simulink model "M"  (R2014a)
settings: Solver=ode45  StartTime=0.0  StopTime=1.0  RelTol=1e-3
undefined symbols (not defined in the file): DiscIntNeverNeededParam, find_system
libraries: powerlib x49, powerlib_extras x39, simulink_extras x4, simulink x2
(part 1 of 4)
settings Model: Creator=HP  LastModifiedBy=HP

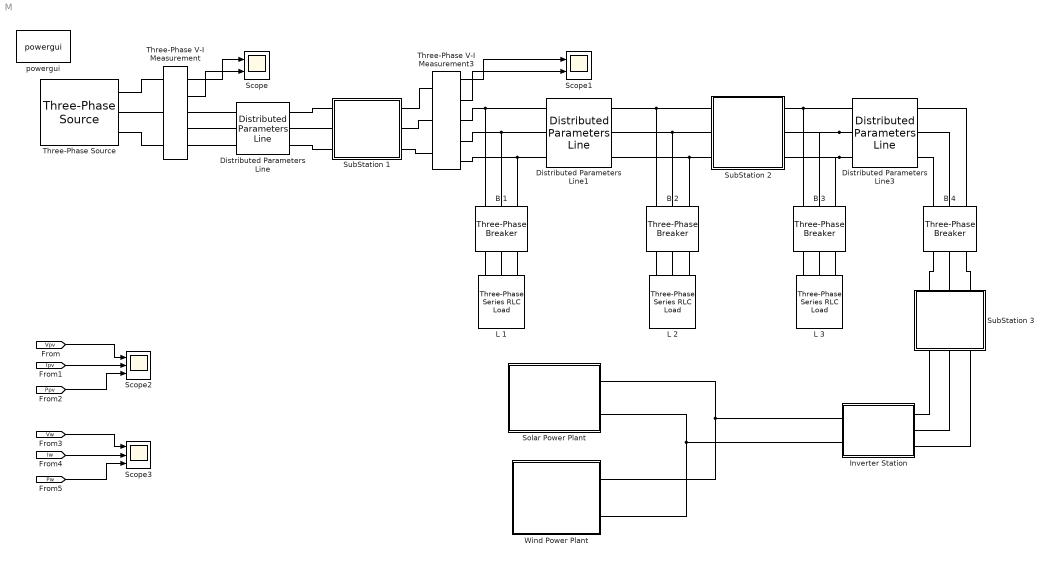
== system M ==
  B 1 : powerlib/Elements/Three-Phase Breaker  InitialState=closed  SwitchA=off  SwitchB=off  SwitchC=off  SwitchTimes="[0.02  0.4]"  External=off  BreakerResistance=0.001  SnubberResistance=1e6  SnubberCapacitance=inf  Measurements=None
  B 2 : powerlib/Elements/Three-Phase Breaker  InitialState=closed  SwitchA=off  SwitchB=off  SwitchC=off  SwitchTimes=[0.001 0.3]  External=off  BreakerResistance=0.001  SnubberResistance=1e6  SnubberCapacitance=inf  Measurements=None
  B 3 : powerlib/Elements/Three-Phase Breaker  InitialState=closed  SwitchA=off  SwitchB=off  SwitchC=off  SwitchTimes="[0.02  0.4]"  External=off  BreakerResistance=0.001  SnubberResistance=1e6  SnubberCapacitance=inf  Measurements=None
  B 4 : powerlib/Elements/Three-Phase Breaker  InitialState=closed  SwitchA=off  SwitchB=off  SwitchC=off  SwitchTimes="[0.001  0.3]"  External=off  BreakerResistance=0.001  SnubberResistance=1e6  SnubberCapacitance=inf  Measurements=None
  Distributed Parameters Line : powerlib/Elements/Distributed Parameters Line  Phases=3  Frequency=50  Resistance=[0.01273 0.3864]  Inductance="[0.9337e-3  4.1264e-3]"  Capacitance=[12.74e-9 7.751e-9]  Length=100  x1=[-0.0006 -7.49436978847816e-10 8343.24139426933 -24001.7141670507;-0.00055 -7.41002543974675e-10 8719.21464973306 -23867.7031951491;-0.0005 -7.32385277811667e-10 9093.03656945038 -23727.8032246242;-0.00045 -7.23587306540276e-10 9464.61491845621 -23582.0487737004;-0.0004 -7.14610800928265e-10 9833.85801535299 -23430.4758051074;-0.00035 -7.05457975794076e-10 10200.6747549317 -23273.1217172073;-0.0003 -6.96131089460354e-10 10564.9746306505 -23110.0253347666;-0.00025 -6.86632443196741e-10 10926.6677569664 -22941.2268993773;-0.0002 -6.76964380652071e-10 11285.6648915124 -22766.7680595275;-0.00015 -6.6712928727611e-10 11641.8774571175 -22586.6918603256;-0.0001 -6.57129589730984e-10 11995.2175636612 -22401.042732879;-5e-05 -6.46967755292433e-10 12345.5980297594 -22209.866483332]  x2=[-0.0006 -3.43708031080569e-09 8376.96946394626 -24147.1732452246;-0.00055 -3.40706257903083e-09 8755.22333035847 -24012.6145509048;-0.0005 -3.37620420554557e-09 9131.31697642113 -23872.131103253;-0.00045 -3.34451280419182e-09 9505.15760665469 -23725.7575644578;-0.0004 -3.31199619434866e-09 9876.65298147754 -23573.5300499998;-0.00035 -3.278662399003e-09 10245.7114399647 -23415.4861197402;-0.0003 -3.24451964277007e-09 10612.241922464 -23251.664768654;-0.00025 -3.20957634986407e-09 10976.1539930633 -23082.1064172082;-0.0002 -3.17384114201967e-09 11337.3578619045 -22906.852901389;-0.00015 -3.13732283636467e-09 11695.7644073378 -22725.947462379;-0.0001 -3.10003044324458e-09 12051.285197911 -22539.4347358883;-5e-05 -3.06197316399936e-09 12403.832514189 -22347.3607411413]  x3=[-0.0006 -1.59881266749975e-11 21.0156321724699 -91.375496743012;-0.00055 -1.62265365289423e-11 22.4483034479498 -91.0341247717012;-0.0005 -1.64609427278014e-11 23.875435940455 -90.6702914922758;-0.00045 -1.66912874353528e-11 25.2966775263978 -90.2840866751534;-0.0004 -1.69175138174866e-11 26.7116775356832 -89.8756056105937;-0.00035 -1.71395660562282e-11 28.1200868382321 -89.4449490851871;-0.0003 -1.73573893635102e-11 29.5215579301236 -88.9922233569873;-0.00025 -1.75709299946909e-11 30.9157450193363 -88.5175401292933;-0.0002 -1.7780135261815e-11 32.3023041110678 -88.0210165230889;-0.00015 -1.7984953546613e-11 33.6808930926096 -87.5027750481441;-0.0001 -1.81853343132381e-11 35.0511718177588 -86.9629435727883;-5e-05 -1.83812281207344e-11 36.412802190744 -86.4016552923603]  x4=[-0.0006 1.01554721594118e-11 30.9066500291586 -89.194818332158;-0.00055 1.0434607945927e-11 32.3038484665578 -88.6983540297173;-0.0005 1.0711169149068e-11 33.6930764127207 -88.1800047356417;-0.00045 1.09850875314961e-11 35.073991096439 -87.6398983448634;-0.0004 1.12562955079492e-11 36.4462517976778 -87.0781681205524;-0.00035 1.15247261619173e-11 37.8095199316424 -86.4949526612362;-0.0003 1.17903132621531e-11 39.1634591323199 -85.8903958666026;-0.00025 1.20529912790137e-11 40.5077353354719 -85.2646469019946;-0.0002 1.2312695400629e-11 41.8420168610601 -84.6178601616057;-0.00015 1.2569361548893e-11 43.1659744950834 -83.9501952303863;-0.0001 1.28229263952743e-11 44.4792815708064 -83.2618168446674;-5e-05 1.3073327376441e-11 45.7816140493595 -82.5528948515154]  x5=0.000565541566995743  V1=ones(3,3)  V2=ones(3,3)  I1=ones(3,3)  I2=ones(3,3)  nHarmo=1  Measurements=None
  Distributed Parameters Line1 : powerlib/Elements/Distributed Parameters Line  Phases=3  Frequency=50  Resistance=[0.01273 0.3864]  Inductance="[0.9337e-3  4.1264e-3]"  Capacitance=[12.74e-9 7.751e-9]  Length=100  x1=[-0.0006 -3.18717949635687e-12 30.305741342475 -96.3292957459078;-0.00055 -1.81472035458282e-12 31.8150774130827 -95.8413899441098;-0.0005 -4.41813457715524e-13 33.3165635893979 -95.3298367134486;-0.00045 9.31202450011464e-13 34.8098294021739 -94.7947622720294;-0.0004 2.30398859746779e-12 36.2945064104155 -94.2362986414639;-0.00035 3.67620627021302e-12 37.7702282922868 -93.6545836142968;-0.0003 5.04751689406933e-12 39.2366309354949 -93.0497607200064;-0.00025 6.41758211865964e-12 40.6933525271301 -92.4219791895918;-0.0002 7.78606390089052e-12 42.1400336429368 -91.7713939187519;-0.00015 9.15262458835922e-12 43.5763173359971 -91.0981654296674;-0.0001 1.05169270026644e-11 45.0018492248011 -90.4024598313942;-5e-05 1.18786345225999e-11 46.416277580686 -89.6844487788787]  x2=[-0.0006 4.51044195495517e-11 -4.09874151767189 -1.70269732982214;-0.00055 4.66840071125865e-11 -4.07149105885821 -1.76686750587743;-0.0005 4.82520760954142e-11 -4.04323602054879 -1.83060173381386;-0.00045 4.98082396004765e-11 -4.01398337425154 -1.89388428816435;-0.0004 5.13521136677142e-11 -3.98374033761921 -1.95669955490553;-0.00035 5.28833173693025e-11 -3.95251437266856 -2.01903203531026;-0.0003 5.44014729036401e-11 -3.92031318393919 -2.08086634977171;-0.00025 5.59062056885653e-11 -3.8871447165926 -2.14218724159802;-0.0002 5.73971444537794e-11 -3.85301715445178 -2.2029795807767;-0.00015 5.88739213324515e-11 -3.81793891798203 -2.26322836770772;-0.0001 6.03361719519841e-11 -3.78191866221331 -2.32291873690442;-5e-05 6.17835355239172e-11 -3.74496527460476 -2.38203596066137]  x3=[-0.0006 -9.52820224818099e-15 3.26026110191264 0.948941267213079;-0.00055 -2.01751092935503e-15 3.24495356999711 1.00003415433087;-0.0005 5.49367818010412e-15 3.22884539434348 1.05088029798491;-0.00045 1.30035118066759e-14 3.21194054940303 1.10146715265009;-0.0004 2.05101370112852e-14 3.19424320619332 1.15178223677695;-0.00035 2.80117016464868e-14 3.17575773126897 1.20181313587138;-0.0003 3.55063548134551e-14 3.15648868564431 1.25154750555764;-0.00025 4.29922473186662e-14 3.13644082366803 1.30097307462422;-0.0002 5.04675321301582e-14 3.11561909185007 1.35007764805151;-0.00015 5.79303648332591e-14 3.09402862764121 1.39884911002079;-0.0001 6.53789040856679e-14 3.07167475816542 1.44727542690361;-5e-05 7.28113120717792e-14 3.04856299890551 1.49534465023088]  x4=[-0.0006 4.21263980623716e-14 -3.18338825813915 -1.31501973217965;-0.00055 3.85890434213476e-14 -3.16234009922532 -1.36485999095589;-0.0005 3.50421675112797e-14 -3.14051168021113 -1.4143634909522;-0.00045 3.14866454707256e-14 -3.11790838693232 -1.46351801792069;-0.0004 2.79233545715464e-14 -3.09453579641331 -1.51231144371734;-0.00035 2.43531740024527e-14 -3.07039967549106 -1.56073172929447;-0.0003 2.07769846520784e-14 -3.04550597939227 -1.60876692767112;-0.00025 1.71956688916338e-14 -3.01986085026394 -1.65640518688086;-0.0002 1.36101103571945e-14 -2.99347061565796 -1.70363475289606;-0.00015 1.00211937316771e-14 -2.96634178696982 -1.75044397252803;-0.0001 6.42980452655666e-15 -2.93848105783208 -1.79682129630222;-5e-05 2.83682886338055e-15 -2.90989530246275 -1.84275528130797]  x5=0.000565541566995743  V1=ones(3,3)  V2=ones(3,3)  I1=ones(3,3)  I2=ones(3,3)  nHarmo=1  Measurements=None
  Distributed Parameters Line3 : powerlib/Elements/Distributed Parameters Line  Phases=3  Frequency=50  Resistance=[0.01273 0.3864]  Inductance="[0.9337e-3  4.1264e-3]"  Capacitance=[12.74e-9 7.751e-9]  Length=100  x1=[-0.0006 2.8165881482916e-13 -0.0164073571497772 -0.00625545726752146;-0.00055 2.89351462434442e-13 -0.0163070765626153 -0.00651240111229207;-0.0005 2.96972716896028e-13 -0.0162027724483196 -0.00676773811953536;-0.00045 3.04520697783418e-13 -0.0160944705423696 -0.0070214052886655;-0.0004 3.1199354274527e-13 -0.0159821975666399 -0.00727334003110421;-0.00035 3.1938940796891e-13 -0.0158659812228075 -0.00752348018572356;-0.0003 3.2670646863526e-13 -0.015745850185516 -0.00777176403418334;-0.00025 3.33942919369088e-13 -0.0156218340953016 -0.00801813031615908;-0.0002 3.41096974684457e-13 -0.0154939635512786 -0.00826251824445717;-0.00015 3.48166869425266e-13 -0.0153622701035905 -0.00850486752001315;-0.0001 3.55150859200777e-13 -0.0152267862456249 -0.00874511834676964;-5e-05 3.62047220816016e-13 -0.0150875454059965 -0.00898321144643007]  x2=[-0.0006 2.80079560694588e-13 -0.016505580431415 -0.00628794373327195;-0.00055 2.87866159152308e-13 -0.0164047774514647 -0.00654642639452007;-0.0005 2.95581730942692e-13 -0.0162999268381482 -0.00680329382301163;-0.00045 3.03224372363849e-13 -0.0161910544617854 -0.00705848264055222;-0.0004 3.10792197708369e-13 -0.0160781871850062 -0.00731192988311961;-0.00035 3.18283339728588e-13 -0.0159613528561221 -0.00756357301639909;-0.0003 3.25695950097306e-13 -0.0158405803022556 -0.00781334995121294;-0.00025 3.33028199863829e-13 -0.0157158993222272 -0.00806119905884;-0.0002 3.40278279905244e-13 -0.0155873406792031 -0.0083070591862216;-0.00015 3.47444401372786e-13 -0.0154549360931048 -0.0085508696710502;-0.0001 3.54524796133211e-13 -0.0153187182327827 -0.00879257035673687;-5e-05 3.61517717205059e-13 -0.0151787207079555 -0.00903210160725407]  x3=[-0.0006 2.67940534806451e-16 -6.28927818269928e-05 -1.6453352061489e-05;-0.00055 2.78631313574821e-16 -6.26265848789131e-05 -1.7439199133093e-05;-0.0005 2.89253344235817e-16 -6.23449357581162e-05 -1.84207433432594e-05;-0.00045 2.99804005962313e-16 -6.20479039573083e-05 -1.93977425106412e-05;-0.0004 3.10280695536402e-16 -6.17355627646417e-05 -2.03699555753132e-05;-0.00035 3.20680827991696e-16 -6.14079892456319e-05 -2.13371426582492e-05;-0.0003 3.31001837251134e-16 -6.10652642241432e-05 -2.22990651205088e-05;-0.00025 3.41241176760117e-16 -6.07074722624464e-05 -2.3255485622118e-05;-0.0002 3.51396320114836e-16 -6.03347016403543e-05 -2.42061681806292e-05;-0.00015 3.61464761685623e-16 -5.99470443334399e-05 -2.51508782293465e-05;-0.0001 3.71444017235176e-16 -5.95445959903431e-05 -2.60893826752014e-05;-5e-05 3.81331624531514e-16 -5.91274559091706e-05 -2.7021449956265e-05]  x4=[-0.0006 3.54343555979096e-16 -6.07615625808273e-05 -2.31395460180172e-05;-0.00055 3.65103703374739e-16 -6.03906063858991e-05 -2.40910924935063e-05;-0.0005 3.75773766894738e-16 -6.00047497124892e-05 -2.50366948524054e-05;-0.00045 3.8635111386058e-16 -5.96040877649581e-05 -2.59761197814818e-05;-0.0004 3.96833134470172e-16 -5.91887194006461e-05 -2.69091354916911e-05;-0.00035 4.07217242441776e-16 -5.87587471054817e-05 -2.78355117753679e-05;-0.0003 4.17500875652129e-16 -5.83142769686952e-05 -2.87550200630258e-05;-0.00025 4.27681496768615e-16 -5.78554186566418e-05 -2.96674334797538e-05;-0.0002 4.37756593875309e-16 -5.73822853857442e-05 -3.05725269011939e-05;-0.00015 4.47723681092757e-16 -5.68949938945571e-05 -3.14700770090878e-05;-0.0001 4.57580299191329e-16 -5.63936644149647e-05 -3.23598623463765e-05;-5e-05 4.67324016197995e-16 -5.58784206425144e-05 -3.32416633718422e-05]  x5=0.000565541566995743  V1=ones(3,3)  V2=ones(3,3)  I1=ones(3,3)  I2=ones(3,3)  nHarmo=1  Measurements=None
  Inverter Station : Subsystem
  L 1 : powerlib/Elements/Three-Phase Series RLC Load  LConnTagsString=A|B|C  Configuration=Y (grounded)  NominalVoltage=254.04  NominalFrequency=50  ActivePower=50e3  InductivePower=100  CapacitivePower=0  Measurements=None  LoadType=constant PQ
  L 2 : powerlib/Elements/Three-Phase Series RLC Load  LConnTagsString=A|B|C  Configuration=Y (grounded)  NominalVoltage=254.04  NominalFrequency=50  ActivePower=50e3  InductivePower=100  CapacitivePower=0  Measurements=None  LoadType=constant PQ
  L 3 : powerlib/Elements/Three-Phase Series RLC Load  LConnTagsString=A|B|C  Configuration=Y (grounded)  NominalVoltage=254.04  NominalFrequency=50  ActivePower=50e3  InductivePower=100  CapacitivePower=0  Measurements=None  LoadType=constant PQ
  Scope : Scope  NumInputPorts=2
      settings: YMin=-25000~-10  YMax=25000~10  SaveName=ScopeData3  MaxDataPoints=100000000
  Scope1 : Scope  NumInputPorts=2
      settings: YMin=-100~-70  YMax=100~70  MaxDataPoints=100000000
  Scope2 : Scope  NumInputPorts=3
      settings: YMin=35~0~0  YMax=90~2.25~140  SaveName=ScopeData4  MaxDataPoints=100000000
  Scope3 : Scope  NumInputPorts=3
      settings: YMin=-100~-5~-5  YMax=1900~5~5  SaveName=ScopeData2  MaxDataPoints=100000000
  Solar Power Plant : Subsystem
  SubStation 1 : Subsystem
  SubStation 2 : Subsystem
  SubStation 3 : Subsystem
  Three-Phase V-I Measurement : powerlib/Measurements/Three-Phase V-I Measurement  VoltageMeasurement=phase-to-ground  SetLabelV=off  LabelV=Vabc_1  Vpu=off  VpuLL=off  CurrentMeasurement=yes  SetLabelI=off  LabelI=Iabc_1  Ipu=off  Pbase=100e6  Vbase=500e3  OutputType=Complex  PhasorSimulation=off  PSBequivalent=0
  Three-Phase V-I Measurement3 : powerlib/Measurements/Three-Phase V-I Measurement  VoltageMeasurement=phase-to-ground  SetLabelV=off  LabelV=Vabc_3  Vpu=off  VpuLL=off  CurrentMeasurement=yes  SetLabelI=off  LabelI=Iabc_3  Ipu=off  Pbase=100e6  Vbase=500e3  OutputType=Complex  PhasorSimulation=off  PSBequivalent=0
  Three-Phase Source : powerlib/Electrical Sources/Three-Phase Source  Voltage=(25000)*1.00008  PhaseAngle=0.13223  Frequency=50  InternalConnection=Yg  SpecifyImpedance=on  Resistance=0.8929  Inductance=16.58e-3  ShortCircuitLevel=100e6  BaseVoltage=63510.4  XRratio=7  BusType=swing  Pref=0  Qref=0  Qmin=-inf  Qmax=inf
  Wind Power Plant : Subsystem
  powergui : powerlib/powergui  Priority=1  SimulationMode=Discrete  SolverType=Tustin  SampleTime=50e-6  frequency=60  SPID=off  DisableSnubberDevices=off  DisableRonSwitches=off  DisableVfSwitches=off  SwTol=0  Interpol=off  DisplayEquations=off  Ts=0  methode=off  frequencyindice=0  Pbase=100e6  ErrMax=0.0001  Iterations=50  UnitsV=kV  UnitsW=MW  FunctionMessages=off  echomessages=off  HookPort=off  EnableUseOfTLC=off  x0status=blocks  RestoreLinks=warning  ResistiveCurrentMeasurement=off  Frange=[0:2:500]  Ylog=off  Xlog=on  ShowGrid=off  save=off  variable=ZData  structure=MLFCDSTAT  ZoomFFT=off  StartTime=0.8  cycles=10  DisplayStyle=1  fundamental=50  FreqAxis=on  MaxFrequency=50000  frequencyindicesteady=1  RmsSteady=1  display=off
  wires:
  Three-Phase V-I Measurement/1 -> Scope/1
  Three-Phase V-I Measurement/2 -> Scope/2
  Three-Phase V-I Measurement3/1 -> Scope1/1
  Three-Phase V-I Measurement3/2 -> Scope1/2
  [Vpv] -> Scope2/1
  [Ppv] -> Scope2/3
  [Ipv] -> Scope2/2
  [Vw] -> Scope3/1
  [Pw] -> Scope3/3
  [Iw] -> Scope3/2
  connections:
  Three-Phase V-I Measurement/LConn2 -- Three-Phase Source/RConn2
  Three-Phase V-I Measurement/LConn1 -- Three-Phase Source/RConn1
  Three-Phase V-I Measurement3/RConn1 -- Distributed Parameters Line1/LConn1 -- B 1/LConn1
  Three-Phase V-I Measurement3/RConn2 -- B 1/LConn2 -- Distributed Parameters Line1/LConn2
  Three-Phase V-I Measurement3/RConn3 -- B 1/LConn3 -- Distributed Parameters Line1/LConn3
  Inverter Station/RConn1 -- SubStation 3/RConn1
  Inverter Station/RConn2 -- SubStation 3/RConn2
  Inverter Station/RConn3 -- SubStation 3/RConn3
  Three-Phase V-I Measurement/RConn1 -- Distributed Parameters Line/LConn1
  Three-Phase V-I Measurement/RConn3 -- Distributed Parameters Line/LConn3
  Three-Phase V-I Measurement/RConn2 -- Distributed Parameters Line/LConn2
  Three-Phase V-I Measurement3/LConn1 -- SubStation 1/RConn1
  SubStation 1/LConn1 -- Distributed Parameters Line/RConn1
  SubStation 1/LConn2 -- Distributed Parameters Line/RConn2
  Three-Phase V-I Measurement3/LConn2 -- SubStation 1/RConn2
  SubStation 1/LConn3 -- Distributed Parameters Line/RConn3
  Three-Phase V-I Measurement3/LConn3 -- SubStation 1/RConn3
  Distributed Parameters Line1/RConn1 -- B 2/LConn1 -- SubStation 2/LConn1
  Distributed Parameters Line1/RConn2 -- B 2/LConn2 -- SubStation 2/LConn2
  Distributed Parameters Line1/RConn3 -- B 2/LConn3 -- SubStation 2/LConn3
  Distributed Parameters Line3/LConn3 -- SubStation 2/RConn3 -- B 3/LConn3
  Distributed Parameters Line3/LConn2 -- SubStation 2/RConn2 -- B 3/LConn2
  B 3/LConn1 -- SubStation 2/RConn1 -- Distributed Parameters Line3/LConn1
  B 4/LConn1 -- Distributed Parameters Line3/RConn3
  B 4/LConn2 -- Distributed Parameters Line3/RConn2
  B 4/LConn3 -- Distributed Parameters Line3/RConn1
  SubStation 3/LConn2 -- B 4/RConn2
  SubStation 3/LConn3 -- B 4/RConn3
  SubStation 3/LConn1 -- B 4/RConn1
  L 1/LConn1 -- B 1/RConn1
  L 1/LConn2 -- B 1/RConn2
  L 1/LConn3 -- B 1/RConn3
  L 2/LConn1 -- B 2/RConn1
  L 2/LConn2 -- B 2/RConn2
  L 2/LConn3 -- B 2/RConn3
  L 3/LConn1 -- B 3/RConn1
  L 3/LConn2 -- B 3/RConn2
  L 3/LConn3 -- B 3/RConn3
  Solar Power Plant/RConn1 -- Wind Power Plant/RConn1 -- Inverter Station/LConn1
  Solar Power Plant/RConn2 -- Wind Power Plant/RConn2 -- Inverter Station/LConn2
  Three-Phase Source/RConn3 -- Three-Phase V-I Measurement/LConn3

== system M/Inverter Station ==
  Constant : Constant  Value=500
  D1 : powerlib/Power Electronics/Diode  Ron=0.001  Lon=0  Vf=0.1  IC=0  UseSnubber=off  Rs=50000  Cs=250e-12  Measurements=off
  D2 : powerlib/Power Electronics/Diode  Ron=0.001  Lon=0  Vf=0.1  IC=0  UseSnubber=off  Rs=50000  Cs=250e-12  Measurements=off
  D3 : powerlib/Power Electronics/Diode  Ron=0.001  Lon=0  Vf=0.1  IC=0  UseSnubber=off  Rs=50000  Cs=250e-12  Measurements=off
  PWM Generator 2 kHz2 : powerlib_extras/Discrete  Control Blocks/Discrete PWM Generator  GeneratorMode="3-arm  bridge (6 pulses)"  Fc=33*50  Ts=1  Internal=off  mIndex=0.4  Freq=60  Phase=0
  Scope4 : Scope  NumInputPorts=2
      settings: ShowLegends=on  YMin=-2.1~-250  YMax=0~4000  SaveName=MLFCDSTAT
  Three-Phase V-I Measurement : powerlib/Measurements/Three-Phase V-I Measurement  VoltageMeasurement=phase-to-ground  SetLabelV=off  LabelV=Vabc  Vpu=off  VpuLL=off  CurrentMeasurement=yes  SetLabelI=off  LabelI=Iabc  Ipu=off  Pbase=100e6  Vbase=500e3  OutputType=Complex  PhasorSimulation=off  PSBequivalent=0
  Unit Delay2 : UnitDelay
  Universal Bridge : powerlib/Power Electronics/Universal Bridge  Arms=3  SnubberResistance=1e5  SnubberCapacitance=inf  Device=MOSFET / Diodes  Ron=1e-3  Lon=0  ForwardVoltages="[  0  0  ]"  ForwardVoltage=0  GTOparameters=[ 10e-6 , 20e-6 ]  IGBTparameters=[ 1e-6 , 2e-6 ]  Measurements=None  Measurements_2=None  converterType=Rectifier
  VSC1 Control : Subsystem  mask(VSC Main Controller){nom=[ 50e3  50 ], Vnom=[ 6350.9 254.03 ], Vnom_dc=500, RLxfo=[0.008  0.04 ], RLchoke=[2e-3*(2*pi*60)/50   2e-3], K_VDCreg=[7  800], K_Ireg=[0.3 20]*1.5, Ts=1}
      mask prompts: nom "Nominal power and frequency [ Pnom(VA)  Fnom(Hz) ]:"; Vnom "Nominal primary and secondary voltages (Vrms LL) [ Vnom_prim   Vnom_sec ]:"; Vnom_dc "Nominal DC bus voltage (V):"; RLxfo "Total transformer leakage impedance (pu/Pnom) [ Rxfo  Lxf ]"; RLchoke "Choke impedance [ R(ohm) L(H) ]"; K_VDCreg "VDC regultator gains [ Kp  Ki ]:"; K_Ireg "Current regulator gains [ Kp  Ki ]:"; Ts "Sample time"
      mask init:
      | Pnom=nom(1);
      | Fnom=nom(2);
      | Vnom_prim=Vnom(1);
      | Vnom_sec=Vnom(2);
      | Zbase=Vnom_sec^2/Pnom;
      | Rtot_pu=RLxfo(1) + RLchoke(1)/Zbase;
      | Ltot_pu=RLxfo(2) + RLchoke(2)/(Zbase/(2*pi*Fnom));
      | Kp_VDCreg=K_VDCreg(1);
      | Ki_VDCreg=K_VDCreg(2);
      | Kp_Ireg=K_Ireg(1);
      | Ki_Ireg=K_Ireg(2);
      | Vdc_ref=Vnom_dc;
      | % Used to determine initial value of Boost Control (MPPT)
      | assignin('base','Vdc_ref_Inv',Vdc_ref);
  R : PMIOPort  Port=1  Side=Right
  + : PMIOPort  Port=2  Side=Left
  - : PMIOPort  Port=3  Side=Left
  Y : PMIOPort  Port=4  Side=Right
  B : PMIOPort  Port=5  Side=Right
  wires:
  [Vabc_5] -> VSC1 Control/1(Vabc_prim)
  [Iabc_5] -> VSC1 Control/2(Iabc_prim)
  PWM Generator 2 kHz2/1 -> Universal Bridge/1
  Constant/1 -> VSC1 Control/3(Vdc_mes)
  Three-Phase V-I Measurement/1 -> Scope4/1
  Three-Phase V-I Measurement/2 -> Scope4/2
  Unit Delay2/1 -> PWM Generator 2 kHz2/1
  VSC1 Control/1(Uref) -> Unit Delay2/1
  connections:
  Universal Bridge/RConn1 -- +/RConn1
  Universal Bridge/RConn2 -- -/RConn1
  Three-Phase V-I Measurement/LConn1 -- Universal Bridge/LConn1
  Three-Phase V-I Measurement/LConn2 -- Universal Bridge/LConn2
  Three-Phase V-I Measurement/RConn2 -- D2/LConn1
  D3/RConn1 -- B/RConn1
  D2/RConn1 -- Y/RConn1
  Three-Phase V-I Measurement/LConn3 -- Universal Bridge/LConn3
  Three-Phase V-I Measurement/RConn1 -- D1/LConn1
  D1/RConn1 -- R/RConn1
  Three-Phase V-I Measurement/RConn3 -- D3/LConn1

== system M/Solar Power Plant ==
  PV array1 : Subsystem
  S1 : Constant  Value=1000
  Step1 : Step  Time=3  After=200  SampleTime=0
  Step3 : Step  Time=2  After=5  SampleTime=0
  Subtract1 : Sum  Inputs=+-
  Subtract3 : Sum
  Tamb1 : Constant  Value=25
  Conn1 : PMIOPort  Port=1  Side=Right
  Conn2 : PMIOPort  Port=2  Side=Right
  wires:
  Subtract3/1 -> PV array1/2(Tamb)
  S1/1 -> Subtract1/1
  Subtract1/1 -> PV array1/1(irradiance)
  Step1/1 -> Subtract1/2
  Tamb1/1 -> Subtract3/1
  Step3/1 -> Subtract3/2
  connections:
  PV array1/RConn1 -- Conn1/RConn1
  PV array1/RConn2 -- Conn2/RConn1

== system M/SubStation 1 ==
  Three-Phase V-I Measurement1 : powerlib/Measurements/Three-Phase V-I Measurement  VoltageMeasurement=phase-to-ground  SetLabelV=on  LabelV=Vabc_2  Vpu=off  VpuLL=off  CurrentMeasurement=yes  SetLabelI=on  LabelI=Iabc_2  Ipu=off  Pbase=100e6  Vbase=500e3  OutputType=Complex  PhasorSimulation=off  PSBequivalent=0
  Three-Phase Breaker1 : powerlib/Elements/Three-Phase Breaker  InitialState=closed  SwitchA=off  SwitchB=off  SwitchC=off  SwitchTimes="[1/50  20/50]"  External=off  BreakerResistance=0.001  SnubberResistance=1e6  SnubberCapacitance=inf  Measurements=None
  Three-Phase Transformer Inductance Matrix Type (Two Windings)1 : powerlib/Elements/Three-Phase Transformer Inductance Matrix Type (Two Windings)  CoreType=Three-limb or five-limb core  Winding1Connection=Yg  Winding2Connection=Yg  AutoTransformer=off  Measurements=None  NominalPower=[100e3 50]  VLLnom=[63510.4 254.03]  WindingResistances=[0.01 0.01]  NoLoadIexcPos=2  NoLoadPlossPos=1000  ShortCircuitReactancePos=0.06  ShortCircuitReactancePosAuto=0.06  NoLoadIexcZero=100  NoLoadPlossZero=1500  ShortCircuitReactanceZero=0.03  ShortCircuitReactanceZeroAuto=0.03
  Conn1 : PMIOPort  Port=1  Side=Right
  Conn2 : PMIOPort  Port=2  Side=Left
  Conn3 : PMIOPort  Port=3  Side=Left
  Conn4 : PMIOPort  Port=4  Side=Right
  Conn5 : PMIOPort  Port=5  Side=Left
  Conn6 : PMIOPort  Port=6  Side=Right
  connections:
  Conn1/RConn1 -- Three-Phase Transformer Inductance Matrix Type (Two Windings)1/RConn1
  Three-Phase V-I Measurement1/LConn3 -- Conn5/RConn1
  Three-Phase V-I Measurement1/LConn2 -- Conn3/RConn1
  Three-Phase V-I Measurement1/LConn1 -- Conn2/RConn1
  Conn6/RConn1 -- Three-Phase Transformer Inductance Matrix Type (Two Windings)1/RConn3
  Conn4/RConn1 -- Three-Phase Transformer Inductance Matrix Type (Two Windings)1/RConn2
  Three-Phase Breaker1/RConn1 -- Three-Phase V-I Measurement1/RConn1
  Three-Phase Breaker1/RConn2 -- Three-Phase V-I Measurement1/RConn2
  Three-Phase Breaker1/RConn3 -- Three-Phase V-I Measurement1/RConn3
  Three-Phase Breaker1/LConn1 -- Three-Phase Transformer Inductance Matrix Type (Two Windings)1/LConn1
  Three-Phase Breaker1/LConn2 -- Three-Phase Transformer Inductance Matrix Type (Two Windings)1/LConn2
  Three-Phase Breaker1/LConn3 -- Three-Phase Transformer Inductance Matrix Type (Two Windings)1/LConn3

== system M/SubStation 2 ==
  Three-Phase V-I Measurement1 : powerlib/Measurements/Three-Phase V-I Measurement  VoltageMeasurement=phase-to-ground  SetLabelV=on  LabelV=Vabc_4  Vpu=off  VpuLL=off  CurrentMeasurement=yes  SetLabelI=on  LabelI=Iabc_4  Ipu=off  Pbase=100e6  Vbase=500e3  OutputType=Complex  PhasorSimulation=off  PSBequivalent=0
  Three-Phase Breaker1 : powerlib/Elements/Three-Phase Breaker  InitialState=closed  SwitchA=off  SwitchB=off  SwitchC=off  SwitchTimes="[1/50  20/50]"  External=off  BreakerResistance=0.001  SnubberResistance=1e6  SnubberCapacitance=inf  Measurements=None
  Three-Phase Transformer Inductance Matrix Type (Two Windings)1 : powerlib/Elements/Three-Phase Transformer Inductance Matrix Type (Two Windings)  CoreType=Three-limb or five-limb core  Winding1Connection=Yg  Winding2Connection=Yg  AutoTransformer=off  Measurements=None  NominalPower=[100e3 50]  VLLnom=[63510.4 254.03]  WindingResistances=[0.01 0.01]  NoLoadIexcPos=2  NoLoadPlossPos=1000  ShortCircuitReactancePos=0.06  ShortCircuitReactancePosAuto=0.06  NoLoadIexcZero=100  NoLoadPlossZero=1500  ShortCircuitReactanceZero=0.03  ShortCircuitReactanceZeroAuto=0.03
  Conn1 : PMIOPort  Port=1  Side=Right
  Conn2 : PMIOPort  Port=2  Side=Left
  Conn3 : PMIOPort  Port=3  Side=Left
  Conn4 : PMIOPort  Port=4  Side=Right
  Conn5 : PMIOPort  Port=5  Side=Left
  Conn6 : PMIOPort  Port=6  Side=Right
  connections:
  Conn1/RConn1 -- Three-Phase Transformer Inductance Matrix Type (Two Windings)1/RConn1
  Three-Phase V-I Measurement1/LConn3 -- Conn5/RConn1
  Three-Phase V-I Measurement1/LConn2 -- Conn3/RConn1
  Three-Phase V-I Measurement1/LConn1 -- Conn2/RConn1
  Conn6/RConn1 -- Three-Phase Transformer Inductance Matrix Type (Two Windings)1/RConn3
  Conn4/RConn1 -- Three-Phase Transformer Inductance Matrix Type (Two Windings)1/RConn2
  Three-Phase Breaker1/RConn1 -- Three-Phase V-I Measurement1/RConn1
  Three-Phase Breaker1/RConn2 -- Three-Phase V-I Measurement1/RConn2
  Three-Phase Breaker1/RConn3 -- Three-Phase V-I Measurement1/RConn3
  Three-Phase Breaker1/LConn1 -- Three-Phase Transformer Inductance Matrix Type (Two Windings)1/LConn1
  Three-Phase Breaker1/LConn2 -- Three-Phase Transformer Inductance Matrix Type (Two Windings)1/LConn2
  Three-Phase Breaker1/LConn3 -- Three-Phase Transformer Inductance Matrix Type (Two Windings)1/LConn3

== system M/SubStation 3 ==
  Three-Phase V-I Measurement1 : powerlib/Measurements/Three-Phase V-I Measurement  VoltageMeasurement=phase-to-ground  SetLabelV=on  LabelV=Vabc_5  Vpu=off  VpuLL=off  CurrentMeasurement=yes  SetLabelI=on  LabelI=Iabc_5  Ipu=off  Pbase=100e6  Vbase=500e3  OutputType=Complex  PhasorSimulation=off  PSBequivalent=0
  Three-Phase Breaker1 : powerlib/Elements/Three-Phase Breaker  InitialState=closed  SwitchA=off  SwitchB=off  SwitchC=off  SwitchTimes="[1/50  20/50]"  External=off  BreakerResistance=0.001  SnubberResistance=1e6  SnubberCapacitance=inf  Measurements=None
  Three-Phase Transformer Inductance Matrix Type (Two Windings)1 : powerlib/Elements/Three-Phase Transformer Inductance Matrix Type (Two Windings)  CoreType=Three-limb or five-limb core  Winding1Connection=Yg  Winding2Connection=Yg  AutoTransformer=off  Measurements=None  NominalPower=[100e3 50]  VLLnom=[63510.4 254.03]  WindingResistances=[0.01 0.01]  NoLoadIexcPos=2  NoLoadPlossPos=1000  ShortCircuitReactancePos=0.06  ShortCircuitReactancePosAuto=0.06  NoLoadIexcZero=100  NoLoadPlossZero=1500  ShortCircuitReactanceZero=0.03  ShortCircuitReactanceZeroAuto=0.03
  Conn1 : PMIOPort  Port=1  Side=Right
  Conn2 : PMIOPort  Port=2  Side=Left
  Conn3 : PMIOPort  Port=3  Side=Left
  Conn4 : PMIOPort  Port=4  Side=Right
  Conn5 : PMIOPort  Port=5  Side=Left
  Conn6 : PMIOPort  Port=6  Side=Right
  connections:
  Conn1/RConn1 -- Three-Phase Transformer Inductance Matrix Type (Two Windings)1/RConn1
  Three-Phase V-I Measurement1/LConn3 -- Conn5/RConn1
  Three-Phase V-I Measurement1/LConn2 -- Conn3/RConn1
  Three-Phase V-I Measurement1/LConn1 -- Conn2/RConn1
  Conn6/RConn1 -- Three-Phase Transformer Inductance Matrix Type (Two Windings)1/RConn3
  Conn4/RConn1 -- Three-Phase Transformer Inductance Matrix Type (Two Windings)1/RConn2
  Three-Phase Breaker1/RConn1 -- Three-Phase V-I Measurement1/RConn1
  Three-Phase Breaker1/RConn2 -- Three-Phase V-I Measurement1/RConn2
  Three-Phase Breaker1/RConn3 -- Three-Phase V-I Measurement1/RConn3
  Three-Phase Breaker1/LConn1 -- Three-Phase Transformer Inductance Matrix Type (Two Windings)1/LConn1
  Three-Phase Breaker1/LConn2 -- Three-Phase Transformer Inductance Matrix Type (Two Windings)1/LConn2
  Three-Phase Breaker1/LConn3 -- Three-Phase Transformer Inductance Matrix Type (Two Windings)1/LConn3

== system M/Wind Power Plant ==
  Bus Selector : BusSelector  OutputSignals=Vdc_V,wr_pu,PQ_pu.P_pu,PQ_pu.Q_pu
  C 2 : powerlib/Elements/Series RLC Branch  LConnTagsString=__new0  RConnTagsString=__new0  BranchType=C  Resistance=1  Inductance=1e-4  SetiL0=off  InitialCurrent=0  Capacitance=3e-4  Setx0=off  InitialVoltage=0  Measurements=None
  CM : powerlib/Measurements/Current Measurement  PhasorSimulation=off  OutputType=Complex  PSBequivalent=0
  Constant1 : Constant  Value=15
  Constant2 : Constant  Value=0
  Divide1 : Product  Inputs=**
  L 2 : powerlib/Elements/Series RLC Branch  LConnTagsString=__new0  RConnTagsString=__new0  BranchType=L  Resistance=1  Inductance=3e-2  SetiL0=off  InitialCurrent=0  Capacitance=1e-6  Setx0=off  InitialVoltage=0  Measurements=None
  PWM Generator : powerlib_extras/Control  Blocks/PWM Generator  GeneratorMode="3-arm  bridge (6 pulses)"  Fc=1080  Internal=on  mIndex=0.4  Freq=50  Phase=0
  Universal Bridge1 : powerlib/Power Electronics/Universal Bridge  Arms=3  SnubberResistance=1e5  SnubberCapacitance=inf  Device=IGBT / Diodes  Ron=1e-3  Lon=0  ForwardVoltages="[  0  0  ]"  ForwardVoltage=0  GTOparameters=[ 10e-6 , 20e-6 ]  IGBTparameters=[ 1e-6 , 2e-6 ]  Measurements=None  Measurements_2=None  converterType=Rectifier
  Voltage Measurement : powerlib/Measurements/Voltage Measurement  PhasorSimulation=off  OutputType=Complex  PSBequivalent=0
  Wind Turbine Type 4 : Subsystem  LoadFcn=%find_system(gcs,'FollowLinks', 'on', 'LookUnderMasks', 'all');  mask(Wind Turbine: Model 7){Nb_wt=1, ShowParameters=Control parameters for 1 wind turbine, nom=[1500/0.9 440 50], Reactances=[ 1.305, 0.296, 0.252, 0.474,  0.243,  0.18 ], Time_constants=[  4.49  0.0681  0.0513  ], Resistance=0.006, mec=[0.62 0.01 1], init=[ 0  0  0  0  0  0  0  0  1 ], Vnom=575, Imax_grid_conv=1.1, RL_grid=[ 0.15 0.15/50], C_var_filter1=150e3, Vdc_nom=1100, C_DClink1=90000e-6, L_R_Boost=[0.0012     5e-3], Pmec1=2e6, wind_speed_CpMax=11, wind0=11, DisplayTurbChar=off, H_WT=4.32, Ksh=0.3, D_mutual=1.5, w_wt0=1, torque0=1, Kdc=[1.1   27.5], Ki_var_reg=0.05, Ki_volt_reg=2, Kgrid_side_cur_reg=[1  50], Kspeed=[5 1], Kboost_cur_reg=[0.025 100], Kp_pitch=15, Kcompensation=[1.5  6], Kfield=[10  20], pitch_max=27, pitch_rate=10, Ts=0.1}
      mask prompts: Nb_wt "Number of wind turbines:"; ShowParameters "Display:"; nom "Nom. power, L-L volt. and freq.: [Pn (VA), Vn (Vrms), fn (Hz)]"; Reactances "Reactances [Xd Xd' Xd'' Xq Xq'' Xl] (p.u.):"; Time_constants "Time constants [Tdo' Tdo'' Tq''] (s):"; Resistance "Resistance Rs (p.u.):"; mec "Inertia constant, friction factor, and pairs of poles: [ H(s)  F(p.u.)  p ]"; init "Initial conditions: [dw(%) th(deg) ia,ib,ic(pu) pha,phb,phc(deg) Vf(pu)]:"; Vnom "Grid-side converter nominal AC voltage (V):"; Imax_grid_conv "Grid-side converter maximum AC current (pu based on generator power and converter nominal AC voltage):"; RL_grid "Grid-side coupling inductor [ L(pu) R(pu),pu based on generator power and converter nominal AC voltage] :"; C_var_filter1 "Line filter capacitor (Q=50) (var):"; Vdc_nom "Nominal DC bus voltage (V)"; C_DClink1 "DC bus capacitor (F):"; L_R_Boost "Boost converter inductance [L(H) R(ohm)]:"; Pmec1 "Nominal mechanical output power (W):"; wind_speed_CpMax "Wind speed at nominal speed and at Cp max (must be between 6 m/s and 30 m/s) (m/s):"; wind0 "Initial wind speed (m/s):"; DisplayTurbChar "Display wind turbine power characteristics:"; H_WT "Wind turbine inertia constant H (s):"; Ksh "Shaft spring constant refer to high-speed shaft (pu of nominal mechanical torque/rad):"; D_mutual "Shaft mutual damping (pu of nominal mechanical torque/pu dw):"; w_wt0 "Turbine initial speed (pu of nominal speed):"; torque0 "Initial output torque (pu of nominal mechanical torque):"; Kdc "DC bus voltage regulator gains [Kp Ki]:"; Ki_var_reg "Grid-side converter var regulator gain [ Ki]:"; Ki_volt_reg "Grid-side converter voltage regulator gain [ Ki]:"; Kgrid_side_cur_reg "Grid-side converter current regulator gains [Kp Ki]:"; Kspeed "Speed regulator gains [Kp Ki]:"; Kboost_cur_reg "Boost inductor current regulator gains [Kp Ki]:"; Kp_pitch "Pitch controller gain [Kp]:"; Kcompensation "Pitch compensation gains [Kp Ki]:"; Kfield "Field excitation gains [Kp Ki]:"; pitch_max "Maximum pitch angle (deg):"; pitch_rate "Maximum rate of change of pitch angle (deg/s)"; Ts "Sample time (s):"
      mask help: This block implements a model of a variable speed pitch controlled wind turbine using a synchronous generator.
      mask init:
      | %Generator data
      | Pnom=nom(1)*Nb_wt;
      | Vnom_gen=nom(2);
      | Fnom=nom(3);
      | Xd=Reactances(1);
      | Xd1=Reactances(2);
      | Xd2=Reactances(3);
      | Xq=Reactances(4);
      | Xq2=Reactances(5);
      | Xl=Reactances(6);
      | Tdo1=Time_constants(1);
      | Tdo2=Time_constants(2);
      | Tq2=Time_constants(3);
      | H=mec(1);
      | F=mec(2);
      | p=mec(3);
      | 
      | % Converters data
      | L_RL=RL_grid(1);
      | R_RL=RL_grid(2);
      | L_Boost=L_R_Boost(1)/Nb_wt;
      | R_Boost=L_R_Boost(2)/Nb_wt;
      | Q_filter=50;
      | C_DClink=C_DClink1*Nb_wt;
      | C_var_filter=C_var_filter1*Nb_wt;
      | 
      | % Controller data
      | Freq_filter=10000;   %Hz
      | Zeta_filter=0.707;
      | Kp_dc=Kdc(1);
      | Ki_dc=Kdc(2);
      | Kp_grid_side_cur_reg=Kgrid_side_cur_reg(1);
      | Ki_grid_side_cur_reg=Kgrid_side_cur_reg(2);
      | Kp_speed=Kspeed(1);
      | Ki_speed=Kspeed(2);
      | Kp_boost_cur_reg=Kboost_cur_reg(1);
      | Ki_boost_cur_reg=Kboost_cur_reg(2);
      | Kp_compensation=Kcompensation(1);
      | Ki_compensation=Kcompensation(2);
      | Kp_field=Kfield(1);
      | Ki_field=Kfield(2);
      | Mod_index_max=1.1;
      | T_speed=5;      %Speed reference time constant (s)
      | Iq_ref_limit_time_constant=0.3; %(s)
      | Current_reg_output_limit=1.1;   %(pu)
      | Var_reg_output_hi_limit=1.1;    %(pu)
      | Var_reg_output_low_limit=0.9;   %(pu)
      | Pitch_time_constant=0.01;       %(s)
      | Vf_limit=10;    %Field voltage limit (pu)
      | Flux_meas_time_constant=1*(1/Fnom); %(s)
      | Freq_sawtooth=2000; %Hz, Boost converter
      | Freq_PWM=3000; %Hz, Inverter
      | Ts_snub=50e-6;  %Sample time to compute snubber resistance
      | 
      | 
      | % Turbine data
      | Pmec=Pmec1*Nb_wt;
      | c1 = 0.6450;
      | c2 = 116;
      | c3 = .4;
      | c4 = 5;
      | c5 = 21;
      | c6 = .00912;  % Set Pmin in stall condition (does not vary with wind_speed_Pmax)
      | c7 = .08;
      | c8 = .035;
      | theta=0;
      | CpMax=.5;
      | lambda_CpMax=9.9495;
      | 
      | c1_c8=[c1 c2 c3 c4 c5 c6 c7 c8];
      |   
      | 
      | %   Cp = c1*(c6*lambda + (-c4 - c3*(2.5 + theta) + c2*(1/(lambda + ...
      | %   c7*(2.5 + theta)) - c8/(1 + (2.5 + theta)^3)))/exp(c5*(1/(lambda + ...
      | %   c7*(2.5 + theta)) - c8/(1 + (2.5 + theta)^3))))
      | 
      | 
      |         %%%%%%%%%%%%%%%%%%%%%%%%%%%%%%%%%%%%%%%%%%%%%%%%%%%%%%%%%%%%%%%%%%%%%%%%%%%
      |         % Operation at Cp max
      |         %%%%%%%%%%%%%%%%%%%%%%%%%%%%%%%%%%%%%%%%%%%%%%%%%%%%%%%%%%%%%%%%%%%%%%%%%%%
      |         
      |         rated_omegar=1;
      |         omegar = rated_omegar;
      |         
      |         % Enforce boundaries on wind speed
      |         % A warning could be displayed
      |         if wind_speed_CpMax < 6
      |             wind_speed_CpMax=6;
      |             disp('Warning: Wind speed at nominal speed and at Cp max has been set to 6 m/s')
      |         end
      |         if wind_speed_CpMax > 30
      |             wind_speed_CpMax=30;
      |             disp('Warning: Wind speed at nominal speed and at Cp max has been set to 30 m/s')
      |         end
      | 
      |         K1=lambda_CpMax/omegar*wind_speed_CpMax;
      |         
      |         % Calculation of K2 needed to get P equal to the requested value at
      |         % Cp max for the requested wind speed
      |         
      |         Prated=Pmec;
      |         P_rated_omegar_theta_zero=0.75;
      |         
      |         K2 = P_rated_omegar_theta_zero*Prated/(wind_speed_CpMax^3*CpMax);
      |         
      |         K1_K2=[K1 K2];
      |         
      |         %%%%%%%%%%%%%%%%%%%%%%%%%%%%%%%%%%%%%%%%%%%%%%%%%%%%%%%%%%%%%%%%%%%%%%%%%%%
      |         % End of calculation for operation at Cp max
      |         %%%%%%%%%%%%%%%%%%%%%%%%%%%%%%%%%%%%%%%%%%%%%%%%%%%%%%%%%%%%%%%%%%%%%%%%%%%
      |         
      | 
      | %%%%%%%%%%%%%%%%%%%%%%%%%%%%%%%%%%%%%%%%%%%%%%%%%%%%%%%%%%%%%%%%%%%%%%%%%%%
      | % Plot turbine characteristics
      | %%%%%%%%%%%%%%%%%%%%%%%%%%%%%%%%%%%%%%%%%%%%%%%%%%%%%%%%%%%%%%%%%%%%%%%%%%% 
      | 
      | DisplayTurbChar=get_param(gcb,'DisplayTurbChar');
      | if strcmp(DisplayTurbChar,'on')
      |     vect_theta = 0:2:30;
      |     
      |     vect_lambda = 1:0.2:30;
      |     
      |     clear Cp;
      |     
      |     for i=1:length(vect_theta)
      |      for j=1:length(vect_lambda)
      |                 Cp(i,j) = c1*(c6*vect_lambda(j) + (-c4 - c3*(2.5 + vect_theta(i)) + c2*(1/(vect_lambda(j) + ...
      |                 c7*(2.5 + vect_theta(i))) - c8/(1 + (2.5 + vect_theta(i))^3)))/exp(c5*(1/(vect_lambda(j) + ...
      |                 c7*(2.5 + vect_theta(i))) - c8/(1 + (2.5 + vect_theta(i))^3))));
      |      end
      |     end
      | 
      |     figure(1);
      |     clf;
      |     hold on;
      | 
      |     plot(vect_lambda, Cp);
      |     axis([0, 25, 0, .6]);
      |     title('Wind Turbine Cp Characteristic (pitch angle increases by step of 2 deg.)');
      |     ylabel('Cp');
      |     set(gca,'ytick',[0 .1 .2 .3 .4 .5 .6]);
      |     xlabel('Lambda');
      |     grid on;
      |     text(10.1,0.51,'Pitch angle 0 degree');
      | 
      |     hold off
      |     
      |     % Plot of the wind turbine mechanical power output (pu) lambda and Cp
      |     % characteristics against wind speed (m/s) for a range of theta.
      |     
      |     wind_speed_range = [1,.2,30];
      |     vect_wind_speed = 1:0.2:30;
      |     
      |     clear lambda;
      |     clear Cp;
      |     clear P;
      | 
      |     for i=1:length(vect_theta)
      |         for j=1:length(vect_wind_speed)
      |             lambda(i,j) = K1*omegar/vect_wind_speed(j);
      |             Cp(i,j) = c1*(c6*lambda(i,j) + (-c4 - c3*(2.5 + vect_theta(i)) + c2*(1/(lambda(i,j) + ...
      |             c7*(2.5 + vect_theta(i))) - c8/(1 + (2.5 + vect_theta(i))^3)))/exp(c5*(1/(lambda(i,j) + ...
      |             c7*(2.5 + vect_theta(i))) - c8/(1 + (2.5 + vect_theta(i))^3))));
      |             P(i,j) = K2/Prated*vect_wind_speed(j)^3*Cp(i,j);
      |         end
      |     end
      |     
      |     
      |     figure(2);
      |     clf;
      |     hold on
      |     
      |     subplot(3,1,1);
      |     plot(vect_wind_speed, P);
      |     axis([0, 35, 0, 1.5]);
      |     title('Wind Turbine Characteristics (w = 1 pu, pitch angle increases by step of 2 deg.)');
      |     ylabel('P (pu)');
      |     set(gca,'ytick',0:.5:4);
      |     grid on;
      |     
      |     subplot(3,1,2);
      |     plot(vect_wind_speed, lambda);
      |     axis([0, 35, 0, 20]);
      |     ylabel('Lambda');
      |     grid on;
      |     
      |     subplot(3,1,3)
      |     plot(vect_wind_speed, Cp);
      |     axis([0, 35, 0, .6]);
      |     xlabel('Wind Speed (m/s)');
      |     ylabel('Cp');
      |     set(gca,'ytick',[0 .1 .2 .3 .4 .5 .6]);
      |     grid on;
      | 
      |     hold off
      |     set_param(gcb,'DisplayTurbChar','off')
      |     
      | end
      mask TypeOptions ShowParameters: Generator data for 1 wind turbine | Converters data for 1 wind turbine | Turbine data for 1 wind turbine | Drive train data for 1 wind turbine | Control parameters for 1 wind turbine
      mask Callback ShowParameters:
      | BlockName=getfullname(gcb);
      | %
      | Param_Show=get_param(BlockName,'ShowParameters');
      | Param_DisplayTurbChar=get_param(BlockName,'DisplayTurbChar');
      | 
      | p_mask{3}='off';p_mask{4}='off';p_mask{5}='off';
      | p_mask{6}='off';p_mask{7}='off';p_mask{8}='off';p_mask{9}='off';
      | p_mask{10}='off';p_mask{11}='off';p_mask{12}='off';p_mask{13}='off';
      | p_mask{14}='off';p_mask{15}='off';p_mask{16}='off';p_mask{17}='off';
      | p_mask{18}='off';p_mask{19}='off';p_mask{20}='off';p_mask{21}='off';
      | p_mask{22}='off';p_mask{23}='off';p_mask{24}='off';p_mask{25}='off';
      | p_mask{26}='off';p_mask{27}='off';p_mask{28}='off';p_mask{29}='off';
      | p_mask{30}='off';p_mask{31}='off';p_mask{32}='off';p_mask{33}='off';
      | p_mask{34}='off';p_mask{35}='off';
      | 
      | switch Param_Show
      | 	case 'Generator data for 1 wind turbine'
      | 		p_mask{3}='on';p_mask{4}='on';p_mask{5}='on';
      |         p_mask{6}='on';p_mask{7}='on';p_mask{8}='on';
      |     case 'Converters data for 1 wind turbine'
      | 		p_mask{9}='on';p_mask{10}='on';p_mask{11}='on';
      |         p_mask{12}='on';p_mask{13}='on';p_mask{14}='on';p_mask{15}='on';
      | 	case 'Turbine data for 1 wind turbine'
      | 		p_mask{16}='on';p_mask{17}='on';p_mask{18}='on';p_mask{19}='on';
      |     case 'Drive train data for 1 wind turbine'
      |         p_mask{20}='on';p_mask{21}='on';p_mask{22}='on';p_mask{23}='on';
      |         p_mask{24}='on';
      |     case 'Control parameters for 1 wind turbine'
      |         p_mask{25}='on';p_mask{26}='on';p_mask{27}='on';
      |         p_mask{28}='on';p_mask{29}='on';p_mask{30}='on';p_mask{31}='on';
      |         p_mask{32}='on';p_mask{33}='on';p_mask{34}='on';p_mask{35}='on';
      | end
      | 
      | ParVisible={'on','on',p_mask{3},p_mask{4},p_mask{5},p_mask{6},...
      |     p_mask{7},p_mask{8},p_mask{9},p_mask{10},p_mask{11},p_mask{12},...
      |     p_mask{13},p_mask{14},p_mask{15},p_mask{16},p_mask{17},p_mask{18},...
      |     p_mask{19},p_mask{20},p_mask{21},p_mask{22},p_mask{23},p_mask{24},...
      |     p_mask{25},p_mask{26},p_mask{27},p_mask{28},p_mask{29},p_mask{30},...
      |     p_mask{31},p_mask{32},p_mask{33},p_mask{34},p_mask{35},'on'};
      | %
      | set_param(BlockName,'MaskVisibilities',ParVisible);
      | set_param(BlockName,'DisplayTurbChar',Param_DisplayTurbChar);
      mask Display: disp(' ');
  Conn1 : PMIOPort  Port=1  Side=Right
  Conn2 : PMIOPort  Port=2  Side=Right
  tag scope: Iw=global, Pw=global, Vw=global
  wires:
  PWM Generator/1 -> Universal Bridge1/1
  Bus Selector/1 -> [Vdc]  "<Vdc_V>"
  Bus Selector/2 -> [wr]  "<wr_pu>"
  Bus Selector/3 -> [P_pu]  "<P_pu>"
  Bus Selector/4 -> [Q_pu]  "<Q_pu>"
  Wind Turbine Type 4/1(m) -> Bus Selector/1
  Constant1/1 -> Wind Turbine Type 4/1("Wind (m/s) ")
  Constant2/1 -> Wind Turbine Type 4/2(Qref_pu)
  CM/1 -> [Iw], Divide1/1
  Voltage Measurement/1 -> [Vw], Divide1/2
  Divide1/1 -> [Pw]
  connections:
  Universal Bridge1/RConn2 -- Conn2/RConn1 -- Voltage Measurement/LConn2 -- C 2/RConn1
  L 2/LConn1 -- Universal Bridge1/RConn1
  L 2/RConn1 -- C 2/LConn1 -- CM/LConn1
  Wind Turbine Type 4/LConn1 -- Universal Bridge1/LConn1
  Wind Turbine Type 4/LConn2 -- Universal Bridge1/LConn2
  Wind Turbine Type 4/LConn3 -- Universal Bridge1/LConn3
  Conn1/RConn1 -- CM/RConn1 -- Voltage Measurement/LConn1

== system M/Inverter Station/VSC1 Control ==
  note: VSC Main Controller
  Vabc_prim : Inport  PortDimensions=3
  Iabc_prim : Inport  Port=2  PortDimensions=3
  Vdc_mes : Inport  Port=3  PortDimensions=1
  Current Regulator : Subsystem
  Gain : Gain  Gain=-1
  Iq_ref : Constant  Value=0
  Mux : Mux  Inputs=2
  PLL & Measurements : Subsystem
  Uabc_ref Generation max (m) = 1 : Subsystem
  VDC Regulator : Subsystem
  Vdc_ref1 : Constant  Value=Vdc_ref
  Uref : Outport
  wires:
  Vdc_ref1/1 -> VDC Regulator/2(Vdc_ref)
  Uabc_ref Generation max (m) = 1/1(Uabc_ref) -> Uref/1
  Iabc_prim/1 -> Gain/1
  Vabc_prim/1 -> PLL & Measurements/1(Vabc_prim)
  Vdc_mes/1 -> VDC Regulator/1(Vdc_mes)
  PLL & Measurements/2(VdVq_prim) -> Current Regulator/1(VdVq_mes)
  PLL & Measurements/3(IdIq_prim) -> Current Regulator/2(IdIq_mes)
  Mux/1 -> Current Regulator/3(IdIq_ref)
  Iq_ref/1 -> Mux/2
  Current Regulator/1(VdVq_conv) -> Uabc_ref Generation max (m) = 1/2(VdVq_conv)
  PLL & Measurements/1(wt) -> Uabc_ref Generation max (m) = 1/1(wt)
  VDC Regulator/1(Id_ref) -> Mux/1
  Gain/1 -> PLL & Measurements/2(Iabc_prim)

== system M/Solar Power Plant/PV array1 ==
  irradiance : Inport
  Tamb : Inport  Port=2
  4700uF : powerlib/Elements/Series RLC Branch  LConnTagsString=__new0  RConnTagsString=__new0  BranchType=C  Resistance=1  Inductance=5e-03  SetiL0=off  InitialCurrent=0  Capacitance=4700e-6  Setx0=off  InitialVoltage=0  Measurements=None
  CCS : powerlib/Electrical Sources/Controlled Current Source  Initialize=on  Source_Type=AC  Amplitude=0  Phase=0  Frequency=0  Measurements=None
  CM : powerlib/Measurements/Current Measurement  PhasorSimulation=off  OutputType=Complex  PSBequivalent=0
  Divide1 : Product  Inputs=**
  Im : Constant  Value=1.93
  Isc : Constant  Value=2.02
  Saturation : Saturate  UpperLimit=100  LowerLimit=0
  Saturation1 : Saturate  UpperLimit=5  LowerLimit=0
  Subsystem1 : Subsystem
  Tref : Constant  Value=55
  VM1 : powerlib/Measurements/Voltage Measurement  PhasorSimulation=off  OutputType=Complex  PSBequivalent=0
  Vm : Constant  Value=70.4
  Voc : Constant  Value=86.8
  + : PMIOPort  Tag=PMCPort  Port=1  Side=Right
  - : PMIOPort  Tag=PMCPort  Port=2  Side=Right
  tag scope: Ipv=global, Ppv=global, Vpv=global
  wires:
  Saturation1/1 -> CCS/1
  CM/1 -> Divide1/2, [Ipv]
  Divide1/1 -> [Ppv]
  Subsystem1/1(Ipv) -> Saturation1/1
  Tref/1 -> Subsystem1/8(Tref)
  VM1/1 -> Divide1/1, [Vpv], Saturation/1
  Saturation/1 -> Subsystem1/1(Vpv)
  Tamb/1 -> Subsystem1/3(Tamb)
  irradiance/1 -> Subsystem1/2(S)
  Vm/1 -> Subsystem1/7(Vm)
  Voc/1 -> Subsystem1/5(Voc)
  Im/1 -> Subsystem1/6(Im)
  Isc/1 -> Subsystem1/4(Isc)
  connections:
  4700uF/RConn1 -- VM1/LConn2 -- CCS/LConn1 -- -/RConn1
  4700uF/LConn1 -- VM1/LConn1 -- CM/RConn1 -- +/RConn1
  CCS/RConn1 -- CM/LConn1
